simulink model "REI_heli"  (R2026a)
settings: Solver=VariableStepAuto  StopTime=30
values from neighbouring files (symbols this model uses):
  A2 = [0 0 -1.49338928581 0 0 0 0 0 1 0 -0.474502630166 0 ... (16 elements, 4x4)]    [REI.mat]
  B2 = [0.118910678044  0; 0.0168  0; -0.00959481287008  0; 0  -0.06]    [REI.mat]
  C2 = [1  0  0  0; 0  1  0  0]    [REI.mat]
  K2 = [43.2819884257  9.37801139417  23.8621675035  1.84697814449; 30.3019399725  -140.497098731  73.036458347  -87.9784869914]    [REI.mat]
  Ki2 = [81.3667639615  11.901849575; 133.141282492  -40.9594567245]    [REI.mat]
libraries: simulink x8, cstblocks_lti x5
settings Model: Creator=victoria  LastModifiedBy=marif

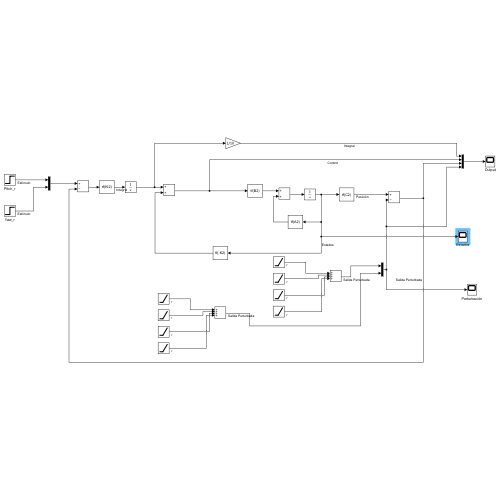
[thumbnail: Simulink's stored preview of the top-level diagram]
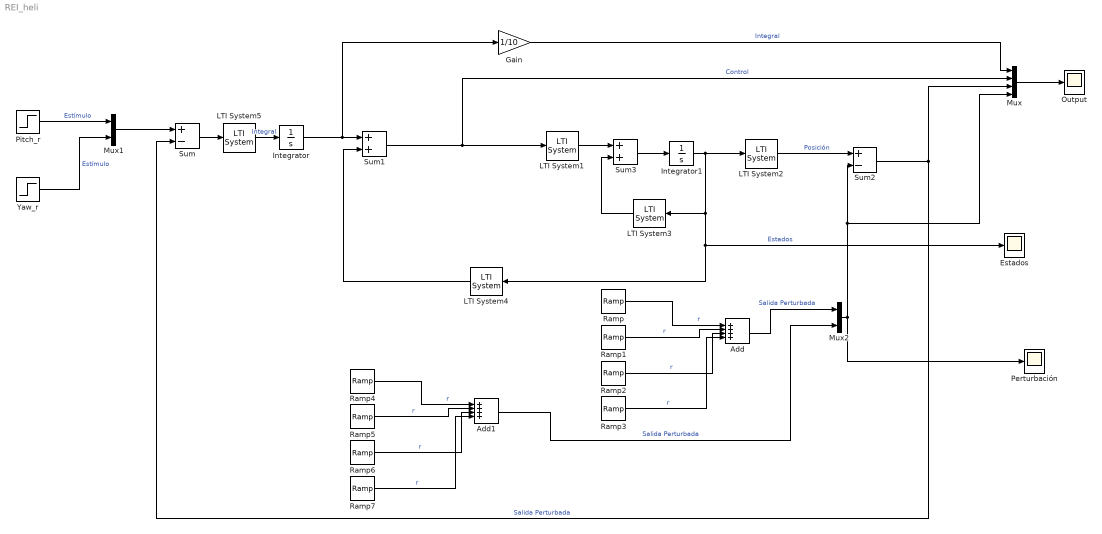
== system REI_heli ==
  Add : Sum  Inputs=++++
  Add1 : Sum  Inputs=++++
  Estados : Scope
      settings: ActiveDisplayYMinimum=-3.2946478151774325  ActiveDisplayYMaximum=3.9485303964821039
  Gain : Gain  Gain=1/10
  Integrator : Integrator
  Integrator1 : Integrator
  LTI System1 : cstblocks_lti/LTI System  sys=tf(B2)  IC=[]  PadeOrder=0
  LTI System2 : cstblocks_lti/LTI System  sys=tf(C2)  IC=[]  PadeOrder=0
  LTI System3 : cstblocks_lti/LTI System  sys=tf(A2)  IC=[]  PadeOrder=0
  LTI System4 : cstblocks_lti/LTI System  sys=tf(-K2)  IC=[]  PadeOrder=0
  LTI System5 : cstblocks_lti/LTI System  sys=tf(Ki2)  IC=[]  PadeOrder=0
  Mux : Mux
  Mux1 : Mux  Inputs=2
  Mux2 : Mux  Inputs=2
  Output : Scope
      settings: ActiveDisplayYMinimum=-3.7412773732936766  ActiveDisplayYMaximum=23.852143110089791
  Perturbación : Scope
      settings: ActiveDisplayYMinimum=-1.39538  ActiveDisplayYMaximum=0.81331
  Pitch_r : Step  Time=0  FinalValue=0.583  SampleTime=0
  Ramp : simulink/Sources/Ramp  slope=0.1  start=11  InitialOutput=0
  Ramp1 : simulink/Sources/Ramp  slope=-0.1  start=12  InitialOutput=0
  Ramp2 : simulink/Sources/Ramp  slope=-0.1  start=15  InitialOutput=0
  Ramp3 : simulink/Sources/Ramp  slope=0.1  start=16  InitialOutput=0
  Ramp4 : simulink/Sources/Ramp  slope=0.35  start=25  InitialOutput=0
  Ramp5 : simulink/Sources/Ramp  slope=-0.35  start=26  InitialOutput=0
  Ramp6 : simulink/Sources/Ramp  slope=-0.35  start=27  InitialOutput=0
  Ramp7 : simulink/Sources/Ramp  slope=0.35  start=28  InitialOutput=0
  Sum : Sum  Inputs=+-
  Sum1 : Sum
  Sum2 : Sum  Inputs=+-
  Sum3 : Sum
  Yaw_r : Step  Time=0  FinalValue=0  SampleTime=0
  wires:
  LTI System1/1 -> Sum3/1
  Sum3/1 -> Integrator1/1
  Integrator1/1 -> LTI System2/1, Estados/1, LTI System4/1, LTI System3/1  "Estados"
  LTI System3/1 -> Sum3/2
  LTI System4/1 -> Sum1/2
  Mux/1 -> Output/1
  LTI System2/1 -> Sum2/1  "Posición"
  Sum1/1 -> LTI System1/1, Mux/2  "Control"
  Sum2/1 -> Mux/3, Sum/2  "Salida Perturbada"
  Gain/1 -> Mux/1  "Integral"
  Pitch_r/1 -> Mux1/1  "Estímulo"
  Yaw_r/1 -> Mux1/2  "Estímulo"
  Mux1/1 -> Sum/1
  Ramp/1 -> Add/1  "r"
  Ramp1/1 -> Add/2  "r"
  Ramp2/1 -> Add/3  "r"
  Ramp3/1 -> Add/4  "r"
  Ramp6/1 -> Add1/3  "r"
  Ramp7/1 -> Add1/4  "r"
  Ramp4/1 -> Add1/1  "r"
  Ramp5/1 -> Add1/2  "r"
  Add1/1 -> Mux2/2  "Salida Perturbada"
  Add/1 -> Mux2/1  "Salida Perturbada"
  Mux2/1 -> Sum2/2, Mux/4, Perturbación/1
  LTI System5/1 -> Integrator/1  "Integral"
  Integrator/1 -> Gain/1, Sum1/1
  Sum/1 -> LTI System5/1
